simulink model "design"  (Simulink 8.4)
settings: Solver=ode23tb  StartTime=0.0  StopTime=1  MaxStep=0.0001  MinStep=0.00001  RelTol=1e-3
libraries: powerlib x63, simulink x12, powerlib_meascontrol x8, RCTblocks x2
settings Model: Creator=SELVA  LastModifiedBy=SELVA  CovSFcnEnable=on
settings DataIOCC: SignalLoggingSaveFormat=Dataset
settings OptimizationCC: ExpressionDepthLimit=128
settings DebuggingCC: UnderspecifiedInitializationDetection=Simplified  MergeDetectMultiDrivingBlocksExec=error  SolverPrmCheckMsg=none  FcnCallInpInsideContextMsg=EnableAllAsError  FrameProcessingCompatibilityMsg=error  StateNameClashWarn=none
settings GRTTargetCC: CombineOutputUpdateFcns=on  GRTInterface=off

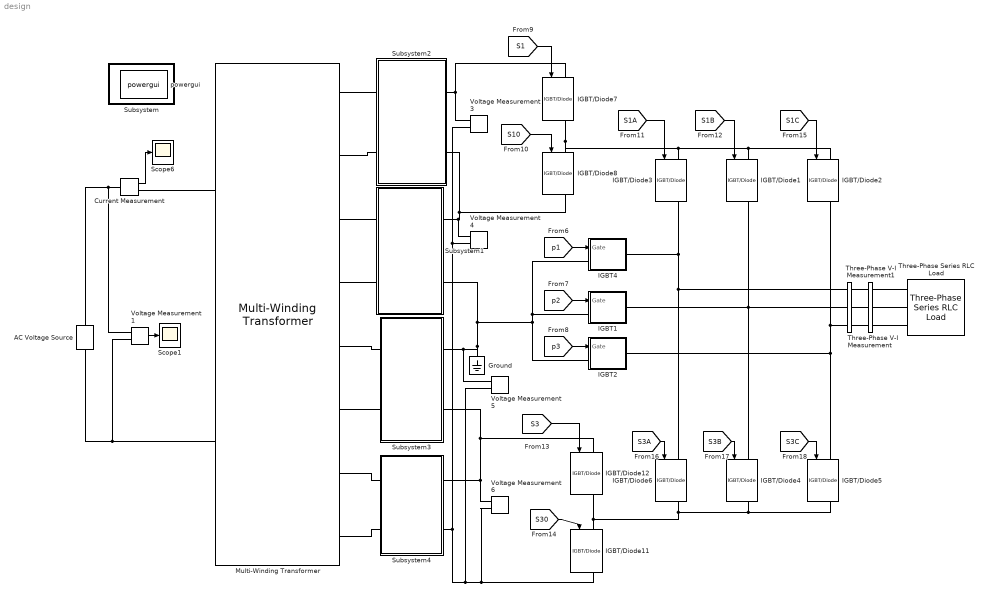
== system design ==
  AC Voltage Source : powerlib/Electrical Sources/AC Voltage Source  Amplitude=325  Phase=0  Frequency=50  SampleTime=0  Measurements=None
  Current Measurement : powerlib/Measurements/Current Measurement  PhasorSimulation=off  OutputType=Complex  PSBequivalent=0
  Ground : powerlib/Elements/Ground  LConnTagsString=a
  IGBT/Diode{1..8,11..12} (10 alike) : powerlib/Power Electronics/IGBT//Diode  Ron=1e-3  Rs=1e5  Cs=inf  Measurements=on
  IGBT1 : Subsystem
  IGBT2 : Subsystem
  IGBT4 : Subsystem
  Multi-Winding Transformer : powerlib/Elements/Multi-Winding Transformer  LeftWindings=1  RightWindings=4  TappedWindings=no taps  NumberOfTaps=2  UNITS=pu  NominalPower=[5000 50]  NominalVoltages="[ 230  115  115 115 115 ]"  WindingResistances="[ 0.005  0.005  0.005  0.005 0.005 ]"  WindingInductances="[ 0.02  0.02  0.02  0.02 0.02 ]"  SetSaturation=on  Rm=50  Lm=50  Saturation=[ 0,0 ; 0.0024,1.2 ; 1.0,1.52 ]  Hysteresis=off  DataFile='hysteresis.mat'  Measurements=Winding currents  MoreParameters=off  BreakLoop=off  DataType=off  InitialFlux=-1.03442051469817  TransfoNumber=1
  Scope1 : Scope
      settings: YMin=3.95  YMax=4.8  SaveName=ScopeData9
  Scope6 : Scope
      settings: YMin=3.95  YMax=4.8  SaveName=ScopeData2
  Subsystem : Subsystem
      mask Display: fprintf('MEASUREMENT \n BLOCK')
  Subsystem1 : Subsystem  mask{r=0, c=1330e-6}
      mask prompts: r "Resistance"; c "Capacitace"
      mask Display: fprintf('Vdc \n RECTIFIER \n WITH \n FILTER')
  Subsystem2 : Subsystem  mask{r=0, c=1330e-6}
      mask prompts: r "Resistance"; c "Capacitace"
      mask Display: fprintf('Vdc \n RECTIFIER \n WITH \n FILTER')
  Subsystem3 : Subsystem  mask{r=0, c=1330e-6}
      mask prompts: r "Resistance"; c "Capacitace"
      mask Display: fprintf('Vdc \n RECTIFIER \n WITH \n FILTER')
  Subsystem4 : Subsystem  mask{r=0, c=1330e-6}
      mask prompts: r "Resistance"; c "Capacitace"
      mask Display: fprintf('Vdc \n RECTIFIER \n WITH \n FILTER')
  Three-Phase Series RLC Load : powerlib/Elements/Three-Phase Series RLC Load  LConnTagsString=A|B|C  Configuration=Y (grounded)  NominalVoltage=400  NominalFrequency=50  ActivePower=500  InductivePower=0  CapacitivePower=0  Measurements=None  LoadType=constant Z
  Three-Phase V-I Measurement : powerlib/Measurements/Three-Phase V-I Measurement  VoltageMeasurement=phase-to-ground  SetLabelV=on  LabelV=Vph  Vpu=off  VpuLL=off  CurrentMeasurement=yes  SetLabelI=on  LabelI=Iab  Ipu=off  Pbase=100e6  Vbase=500e3  OutputType=Complex  PhasorSimulation=off  PSBequivalent=0
  Three-Phase V-I Measurement1 : powerlib/Measurements/Three-Phase V-I Measurement  VoltageMeasurement=phase-to-phase  SetLabelV=on  LabelV=Vl  Vpu=off  VpuLL=off  CurrentMeasurement=yes  SetLabelI=on  LabelI=Iabc  Ipu=off  Pbase=100e6  Vbase=500e3  OutputType=Complex  PhasorSimulation=off  PSBequivalent=0
  Voltage Measurement{1,3..6} (5 alike) : powerlib/Measurements/Voltage Measurement  PhasorSimulation=off  OutputType=Complex  PSBequivalent=0
  powergui : powerlib/powergui  Priority=1  SimulationMode=Discrete  SolverType=Tustin/Backward Euler (TBE)  SampleTime=50e-6  frequency=60  SPID=off  DisableSnubberDevices=off  DisableRonSwitches=off  DisableVfSwitches=off  SwTol=0  DisplayEquations=off  Interpol=off  methode=off  Ts=100  frequencyindice=0  Pbase=100e6  ErrMax=1e-4  Iterations=50  UnitsV=kV  UnitsW=MW  FunctionMessages=off  echomessages=off  HookPort=off  EnableUseOfTLC=off  x0status=blocks  RestoreLinks=warning  ResistiveCurrentMeasurement=off  Frange=[0:2:500]  Ylog=off  Xlog=off  ShowGrid=off  save=off  variable=ZData  structure=ScopeData1  ZoomFFT=off  StartTime=0.5  cycles=1  DisplayStyle=1  fundamental=50  FreqAxis=off  MaxFrequency=1000  frequencyindicesteady=1  RmsSteady=1  display=off
  wires:
  [S3C] -> IGBT/Diode5/1
  [S1A] -> IGBT/Diode3/1
  [S1B] -> IGBT/Diode1/1
  [S1C] -> IGBT/Diode2/1
  [S3A] -> IGBT/Diode6/1
  [S3B] -> IGBT/Diode4/1
  Current Measurement/1 -> Scope6/1
  [S3] -> IGBT/Diode12/1
  [p2] -> IGBT1/1(Gate)
  [p3] -> IGBT2/1(Gate)
  [p1] -> IGBT4/1(Gate)
  [S10] -> IGBT/Diode8/1
  [S1] -> IGBT/Diode7/1
  [S30] -> IGBT/Diode11/1
  Voltage Measurement1/1 -> Scope1/1
  connections:
  Three-Phase V-I Measurement/LConn1 -- IGBT4/RConn1 -- IGBT/Diode3/RConn1 -- IGBT/Diode6/LConn1
  IGBT/Diode3/LConn1 -- IGBT/Diode7/RConn1 -- IGBT/Diode8/LConn1 -- IGBT/Diode2/LConn1 -- IGBT/Diode1/LConn1
  Three-Phase V-I Measurement1/LConn2 -- Three-Phase V-I Measurement/RConn2
  Three-Phase V-I Measurement1/LConn1 -- Three-Phase V-I Measurement/RConn1
  Three-Phase V-I Measurement1/LConn3 -- Three-Phase V-I Measurement/RConn3
  Three-Phase Series RLC Load/LConn2 -- Three-Phase V-I Measurement1/RConn2
  Three-Phase Series RLC Load/LConn1 -- Three-Phase V-I Measurement1/RConn1
  Three-Phase V-I Measurement1/RConn3 -- Three-Phase Series RLC Load/LConn3
  Subsystem2/LConn2 -- Multi-Winding Transformer/RConn2
  Subsystem1/LConn2 -- Multi-Winding Transformer/RConn4
  Subsystem3/LConn1 -- Multi-Winding Transformer/RConn5
  Subsystem1/LConn1 -- Multi-Winding Transformer/RConn3
  Subsystem3/LConn2 -- Multi-Winding Transformer/RConn6
  Subsystem2/LConn1 -- Multi-Winding Transformer/RConn1
  AC Voltage Source/LConn1 -- Voltage Measurement1/LConn2 -- Multi-Winding Transformer/LConn2
  Current Measurement/LConn1 -- Voltage Measurement1/LConn1 -- AC Voltage Source/RConn1
  Current Measurement/RConn1 -- Multi-Winding Transformer/LConn1
  IGBT/Diode4/RConn1 -- IGBT/Diode11/LConn1 -- IGBT/Diode12/RConn1 -- IGBT/Diode6/RConn1 -- IGBT/Diode5/RConn1
  IGBT/Diode12/LConn1 -- Voltage Measurement6/LConn1 -- Subsystem4/RConn1 -- Subsystem3/RConn2
  Subsystem2/RConn2 -- Voltage Measurement4/LConn1 -- Subsystem1/RConn1 -- IGBT/Diode8/RConn1
  IGBT/Diode2/RConn1 -- IGBT/Diode5/LConn1 -- IGBT2/RConn1 -- Three-Phase V-I Measurement/LConn3
  Three-Phase V-I Measurement/LConn2 -- IGBT/Diode4/LConn1 -- IGBT1/RConn1 -- IGBT/Diode1/RConn1
  Subsystem4/RConn2 -- Voltage Measurement4/LConn2 -- Voltage Measurement3/LConn2 -- Voltage Measurement5/LConn2 -- Voltage Measurement6/LConn2 -- IGBT/Diode11/RConn1
  Subsystem2/RConn1 -- Voltage Measurement3/LConn1 -- IGBT/Diode7/LConn1
  Multi-Winding Transformer/RConn8 -- Subsystem4/LConn2
  Multi-Winding Transformer/RConn7 -- Subsystem4/LConn1
  IGBT4/LConn1 -- IGBT1/LConn1 -- IGBT2/LConn1 -- Voltage Measurement5/LConn1 -- Subsystem3/RConn1 -- Ground/LConn1 -- Subsystem1/RConn2

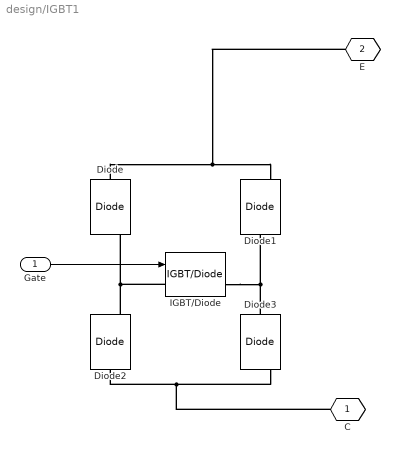
== system design/IGBT1 ==
  Gate : Inport
  Diode{,1..3} (4 alike) : powerlib/Power Electronics/Diode  Ron=0.001  Lon=0  Vf=0.8  IC=0  UseSnubber=off  Rs=500  Cs=250e-9  Measurements=on
  IGBT/Diode : powerlib/Power Electronics/IGBT//Diode  Ron=1e-3  Rs=1e5  Cs=inf  Measurements=on
  C : PMIOPort  Port=1  Side=Left
  E : PMIOPort  Port=2  Side=Right
  wires:
  Gate/1 -> IGBT/Diode/1
  connections:
  E/RConn1 -- Diode/LConn1 -- Diode1/RConn1
  C/RConn1 -- Diode3/RConn1 -- Diode2/LConn1
  IGBT/Diode/RConn1 -- Diode3/LConn1 -- Diode1/LConn1
  IGBT/Diode/LConn1 -- Diode2/RConn1 -- Diode/RConn1

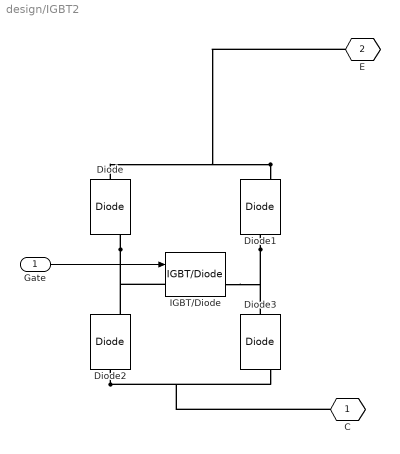
== system design/IGBT2 ==
  Gate : Inport
  Diode{,1..3} (4 alike) : powerlib/Power Electronics/Diode  Ron=0.001  Lon=0  Vf=0.8  IC=0  UseSnubber=off  Rs=500  Cs=250e-9  Measurements=on
  IGBT/Diode : powerlib/Power Electronics/IGBT//Diode  Ron=1e-3  Rs=1e5  Cs=inf  Measurements=on
  C : PMIOPort  Port=1  Side=Left
  E : PMIOPort  Port=2  Side=Right
  wires:
  Gate/1 -> IGBT/Diode/1
  connections:
  Diode/RConn1 -- Diode2/RConn1 -- IGBT/Diode/LConn1
  Diode1/LConn1 -- Diode3/LConn1 -- IGBT/Diode/RConn1
  Diode2/LConn1 -- Diode3/RConn1 -- C/RConn1
  Diode1/RConn1 -- Diode/LConn1 -- E/RConn1

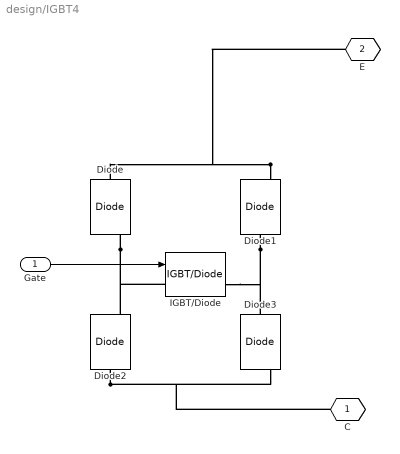
== system design/IGBT4 ==
  Gate : Inport
  Diode{,1..3} (4 alike) : powerlib/Power Electronics/Diode  Ron=0.001  Lon=0  Vf=0.8  IC=0  UseSnubber=off  Rs=500  Cs=250e-9  Measurements=on
  IGBT/Diode : powerlib/Power Electronics/IGBT//Diode  Ron=1e-3  Rs=1e5  Cs=inf  Measurements=on
  C : PMIOPort  Port=1  Side=Left
  E : PMIOPort  Port=2  Side=Right
  wires:
  Gate/1 -> IGBT/Diode/1
  connections:
  Diode/RConn1 -- Diode2/RConn1 -- IGBT/Diode/LConn1
  Diode1/LConn1 -- Diode3/LConn1 -- IGBT/Diode/RConn1
  Diode2/LConn1 -- Diode3/RConn1 -- C/RConn1
  Diode1/RConn1 -- Diode/LConn1 -- E/RConn1

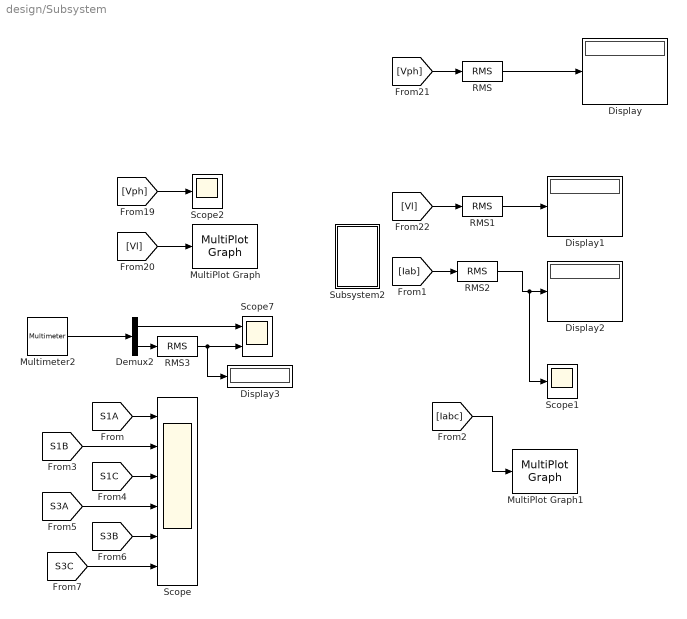
== system design/Subsystem ==
  Demux2 : Demux  Outputs=2
  Display{,1..3} (4 alike) : Display
  MultiPlot Graph : RCTblocks/MultiPlot Graph  Tag=MultiPlot  tmin=0  tmax=20  ymin=-1  ymax=1  Tsamp=-1  vnamesave=multisimout
  MultiPlot Graph1 : RCTblocks/MultiPlot Graph  Tag=MultiPlot  tmin=0  tmax=20  ymin=-1  ymax=1  Tsamp=-1  vnamesave=multisimout1
  Multimeter2 : powerlib/Measurements/Multimeter  PhasorSimulation=off  OutputType=Complex  sel=[11 10]  L=14  Gain=[1 1]  yselected={'I_RightWinding_1: Multi-Winding Transformer','I_LeftWinding_1: Multi-Winding Transformer'};  PSBOutputType=1  PSBequivalent=0  AxesSetting=[0,0.1,-100,100]  Display=0  SavedBlockNames=-11
  RMS{,1..3} (4 alike) : powerlib_meascontrol/Measurements/RMS  TrueRMS=on  Freq=50  RMSInit=0  Ts=0
  Scope : Scope  NumInputPorts=6
      settings: TimeRange=1  YMin=0.7416015625000001~0~0~0~0~0  YMax=0.8755859375~1~1~1~1~1  SaveName=ScopeData7
  Scope1 : Scope
      settings: YMin=0.968  YMax=0.987
  Scope2 : Scope
      settings: YMin=-350  YMax=350
  Scope7 : Scope  NumInputPorts=2
      settings: YMin=-175~-350  YMax=175~350  SaveName=ScopeData6
  Subsystem2 : Subsystem  mask{fc=1000, m=1}
      mask prompts: fc "Switching frequency"; m "modulation index"
  wires:
  [Vph] -> Scope2/1
  [Vl] -> MultiPlot Graph/1
  RMS/1 -> Display/1
  [Vph] -> RMS/1
  RMS1/1 -> Display1/1
  [Vl] -> RMS1/1
  [Iab] -> RMS2/1
  RMS2/1 -> Scope1/1, Display2/1
  [Iabc] -> MultiPlot Graph1/1
  Multimeter2/1 -> Demux2/1
  Demux2/1 -> Scope7/1
  [S1A] -> Scope/1
  [S1B] -> Scope/2
  [S1C] -> Scope/3
  [S3A] -> Scope/4
  [S3B] -> Scope/5
  [S3C] -> Scope/6
  Demux2/2 -> RMS3/1
  RMS3/1 -> Display3/1, Scope7/2

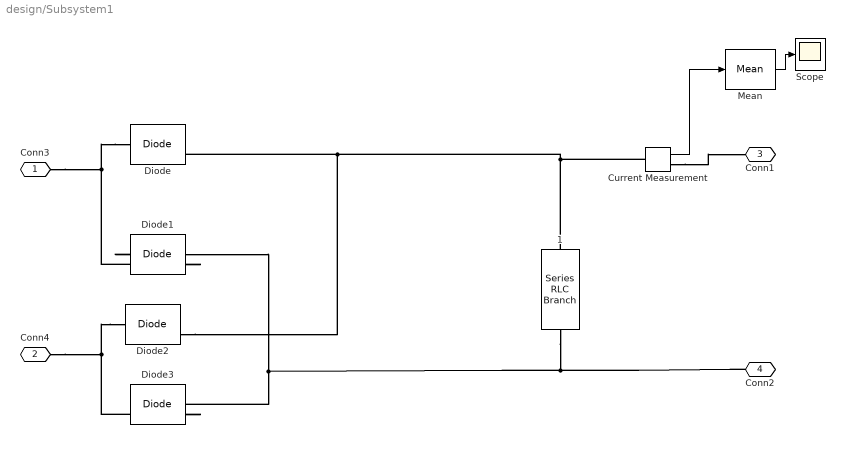
== system design/Subsystem1 ==
  1 : powerlib/Elements/Series RLC Branch  LConnTagsString=__new0  RConnTagsString=__new0  BranchType=C  Resistance=r  Inductance=1e-3  SetiL0=off  InitialCurrent=0  Capacitance=c  Setx0=off  InitialVoltage=0  Measurements=Branch voltage and current
  Current Measurement : powerlib/Measurements/Current Measurement  PhasorSimulation=off  OutputType=Complex  PSBequivalent=0
  Diode{,1..3} (4 alike) : powerlib/Power Electronics/Diode  Ron=0.001  Lon=0  Vf=0.8  IC=0  UseSnubber=off  Rs=500  Cs=250e-9  Measurements=on
  Mean : powerlib_meascontrol/Measurements/Mean  Freq=50  Vinit=0  Ts=0
  Scope : Scope
      settings: YMin=0.6175  YMax=0.67  SaveName=ScopeData8
  Conn3 : PMIOPort  Port=1  Side=Left
  Conn4 : PMIOPort  Port=2  Side=Left
  Conn1 : PMIOPort  Port=3  Side=Right
  Conn2 : PMIOPort  Port=4  Side=Right
  wires:
  Mean/1 -> Scope/1
  Current Measurement/1 -> Mean/1
  connections:
  Current Measurement/RConn1 -- Conn1/RConn1
  Diode/RConn1 -- 1/LConn1 -- Current Measurement/LConn1 -- Diode2/RConn1
  Diode2/LConn1 -- Conn4/RConn1 -- Diode3/RConn1
  Diode/LConn1 -- Conn3/RConn1 -- Diode1/RConn1
  Diode1/LConn1 -- 1/RConn1 -- Conn2/RConn1 -- Diode3/LConn1

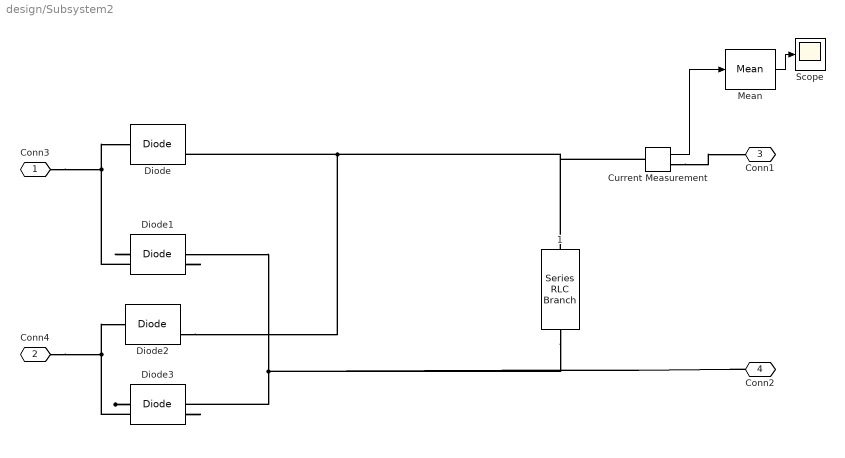
== system design/Subsystem2 ==
  1 : powerlib/Elements/Series RLC Branch  LConnTagsString=__new0  RConnTagsString=__new0  BranchType=C  Resistance=r  Inductance=1e-3  SetiL0=off  InitialCurrent=0  Capacitance=c  Setx0=off  InitialVoltage=0  Measurements=Branch voltage and current
  Current Measurement : powerlib/Measurements/Current Measurement  PhasorSimulation=off  OutputType=Complex  PSBequivalent=0
  Diode{,1..3} (4 alike) : powerlib/Power Electronics/Diode  Ron=0.001  Lon=0  Vf=0.8  IC=0  UseSnubber=off  Rs=500  Cs=250e-9  Measurements=on
  Mean : powerlib_meascontrol/Measurements/Mean  Freq=50  Vinit=0  Ts=0
  Scope : Scope
      settings: YMin=0.6175  YMax=0.67  SaveName=ScopeData8
  Conn3 : PMIOPort  Port=1  Side=Left
  Conn4 : PMIOPort  Port=2  Side=Left
  Conn1 : PMIOPort  Port=3  Side=Right
  Conn2 : PMIOPort  Port=4  Side=Right
  wires:
  Current Measurement/1 -> Mean/1
  Mean/1 -> Scope/1
  connections:
  Diode3/LConn1 -- Conn2/RConn1 -- 1/RConn1 -- Diode1/LConn1
  Diode1/RConn1 -- Conn3/RConn1 -- Diode/LConn1
  Diode3/RConn1 -- Conn4/RConn1 -- Diode2/LConn1
  Diode2/RConn1 -- Current Measurement/LConn1 -- 1/LConn1 -- Diode/RConn1
  Current Measurement/RConn1 -- Conn1/RConn1

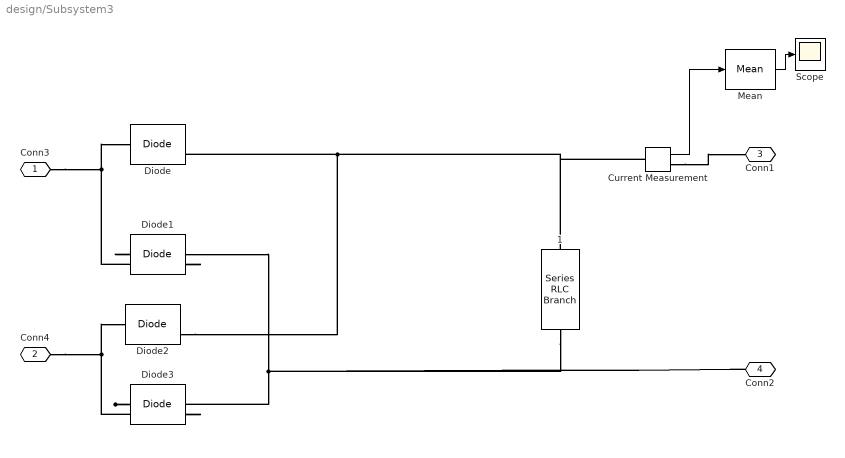
== system design/Subsystem3 ==
  1 : powerlib/Elements/Series RLC Branch  LConnTagsString=__new0  RConnTagsString=__new0  BranchType=C  Resistance=r  Inductance=1e-3  SetiL0=off  InitialCurrent=0  Capacitance=c  Setx0=off  InitialVoltage=0  Measurements=Branch voltage and current
  Current Measurement : powerlib/Measurements/Current Measurement  PhasorSimulation=off  OutputType=Complex  PSBequivalent=0
  Diode{,1..3} (4 alike) : powerlib/Power Electronics/Diode  Ron=0.001  Lon=0  Vf=0.8  IC=0  UseSnubber=off  Rs=500  Cs=250e-9  Measurements=on
  Mean : powerlib_meascontrol/Measurements/Mean  Freq=50  Vinit=0  Ts=0
  Scope : Scope
      settings: YMin=0.6175  YMax=0.67  SaveName=ScopeData8
  Conn3 : PMIOPort  Port=1  Side=Left
  Conn4 : PMIOPort  Port=2  Side=Left
  Conn1 : PMIOPort  Port=3  Side=Right
  Conn2 : PMIOPort  Port=4  Side=Right
  wires:
  Current Measurement/1 -> Mean/1
  Mean/1 -> Scope/1
  connections:
  Diode3/LConn1 -- Conn2/RConn1 -- 1/RConn1 -- Diode1/LConn1
  Diode1/RConn1 -- Conn3/RConn1 -- Diode/LConn1
  Diode3/RConn1 -- Conn4/RConn1 -- Diode2/LConn1
  Diode2/RConn1 -- Current Measurement/LConn1 -- 1/LConn1 -- Diode/RConn1
  Current Measurement/RConn1 -- Conn1/RConn1

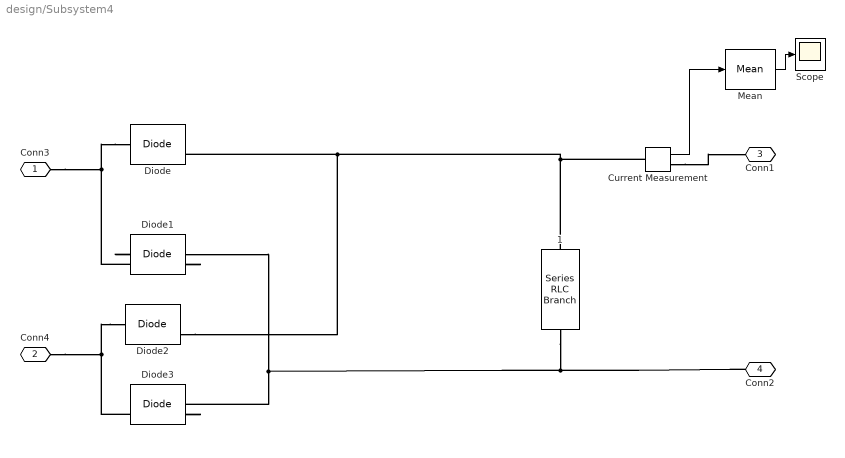
== system design/Subsystem4 ==
  1 : powerlib/Elements/Series RLC Branch  LConnTagsString=__new0  RConnTagsString=__new0  BranchType=C  Resistance=r  Inductance=1e-3  SetiL0=off  InitialCurrent=0  Capacitance=c  Setx0=off  InitialVoltage=0  Measurements=Branch voltage and current
  Current Measurement : powerlib/Measurements/Current Measurement  PhasorSimulation=off  OutputType=Complex  PSBequivalent=0
  Diode{,1..3} (4 alike) : powerlib/Power Electronics/Diode  Ron=0.001  Lon=0  Vf=0.8  IC=0  UseSnubber=off  Rs=500  Cs=250e-9  Measurements=on
  Mean : powerlib_meascontrol/Measurements/Mean  Freq=50  Vinit=0  Ts=0
  Scope : Scope
      settings: YMin=0.6175  YMax=0.67  SaveName=ScopeData8
  Conn3 : PMIOPort  Port=1  Side=Left
  Conn4 : PMIOPort  Port=2  Side=Left
  Conn1 : PMIOPort  Port=3  Side=Right
  Conn2 : PMIOPort  Port=4  Side=Right
  wires:
  Mean/1 -> Scope/1
  Current Measurement/1 -> Mean/1
  connections:
  Current Measurement/RConn1 -- Conn1/RConn1
  Diode/RConn1 -- 1/LConn1 -- Current Measurement/LConn1 -- Diode2/RConn1
  Diode2/LConn1 -- Conn4/RConn1 -- Diode3/RConn1
  Diode/LConn1 -- Conn3/RConn1 -- Diode1/RConn1
  Diode1/LConn1 -- 1/RConn1 -- Conn2/RConn1 -- Diode3/LConn1

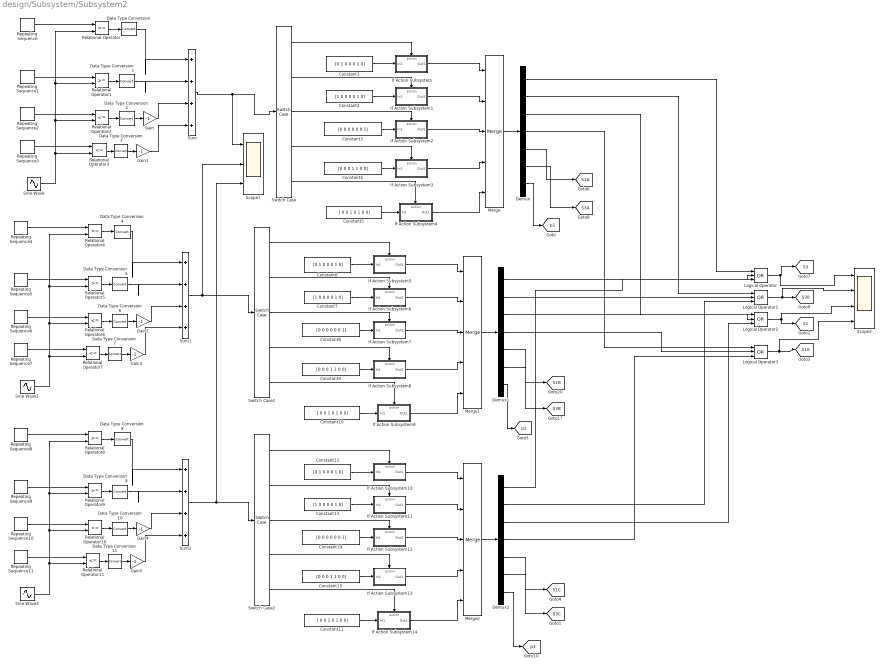
== system design/Subsystem/Subsystem2 ==
  Constant1 : Constant  Value=[0 1 0 0 0 1 0]
  Constant10 : Constant  Value=[ 0 0 1 0 1 0 0]
  Constant11 : Constant  Value=[ 0 0 1 0 1 0 0]
  Constant12 : Constant  Value=[0 1 0 0 0 1 0]
  Constant13 : Constant  Value=[1 0 0 0 0 1 0]
  Constant14 : Constant  Value=[0 0 0 0 0 0 1]
  Constant15 : Constant  Value=[0 0 0 1 1 0 0]
  Constant2 : Constant  Value=[1 0 0 0 0 1 0]
  Constant3 : Constant  Value=[0 0 0 0 0 0 1]
  Constant4 : Constant  Value=[0 0 0 1 1 0 0]
  Constant5 : Constant  Value=[ 0 0 1 0 1 0 0]
  Constant6 : Constant  Value=[0 1 0 0 0 1 0]
  Constant7 : Constant  Value=[1 0 0 0 0 1 0]
  Constant8 : Constant  Value=[0 0 0 0 0 0 1]
  Constant9 : Constant  Value=[0 0 0 1 1 0 0]
  Data Type Conversion{,1..11} (12 alike) : DataTypeConversion
  Demux : Demux  Outputs=7
  Demux1 : Demux  Outputs=7
  Demux2 : Demux  Outputs=7
  Gain{,1..5} (6 alike) : Gain  Gain=-1
  If Action Subsystem : Subsystem  TreatAsAtomicUnit=on
  If Action Subsystem1 : Subsystem  TreatAsAtomicUnit=on
  If Action Subsystem10 : Subsystem  TreatAsAtomicUnit=on
  If Action Subsystem11 : Subsystem  TreatAsAtomicUnit=on
  If Action Subsystem12 : Subsystem  TreatAsAtomicUnit=on
  If Action Subsystem13 : Subsystem  TreatAsAtomicUnit=on
  If Action Subsystem14 : Subsystem  TreatAsAtomicUnit=on
  If Action Subsystem2 : Subsystem  TreatAsAtomicUnit=on
  If Action Subsystem3 : Subsystem  TreatAsAtomicUnit=on
  If Action Subsystem4 : Subsystem  TreatAsAtomicUnit=on
  If Action Subsystem5 : Subsystem  TreatAsAtomicUnit=on
  If Action Subsystem6 : Subsystem  TreatAsAtomicUnit=on
  If Action Subsystem7 : Subsystem  TreatAsAtomicUnit=on
  If Action Subsystem8 : Subsystem  TreatAsAtomicUnit=on
  If Action Subsystem9 : Subsystem  TreatAsAtomicUnit=on
  Logical Operator{,1..3} (4 alike) : Logic  Operator=OR  Inputs=3  AllPortsSameDT=off  OutDataTypeStr=boolean
  Merge : Merge  Inputs=5
  Merge1 : Merge  Inputs=5
  Merge2 : Merge  Inputs=5
  Relational Operator{,1,4..5,8..9} (6 alike) : RelationalOperator  OutDataTypeStr=boolean
  Relational Operator{2..3,6..7,10..11} (6 alike) : RelationalOperator  Operator=<=  OutDataTypeStr=boolean
  Repeating Sequence : simulink/Sources/Repeating Sequence  rep_seq_t="[0 (1/fc)/2  (1/fc)]"  rep_seq_y=[1 2 1]
  Repeating Sequence1 : simulink/Sources/Repeating Sequence  rep_seq_t="[0 (1/fc)/2  (1/fc)]"  rep_seq_y=[1 0 1]
  Repeating Sequence10 : simulink/Sources/Repeating Sequence  rep_seq_t="[0 (1/fc)/2  (1/fc)]"  rep_seq_y=[-1 0 -1]
  Repeating Sequence11 : simulink/Sources/Repeating Sequence  rep_seq_t="[0 (1/fc)/2  (1/fc)]"  rep_seq_y=[-1 -2 -1]
  Repeating Sequence2 : simulink/Sources/Repeating Sequence  rep_seq_t="[0 (1/fc)/2  (1/fc)]"  rep_seq_y=[-1 0 -1]
  Repeating Sequence3 : simulink/Sources/Repeating Sequence  rep_seq_t="[0 (1/fc)/2  (1/fc)]"  rep_seq_y=[-1 -2 -1]
  Repeating Sequence4 : simulink/Sources/Repeating Sequence  rep_seq_t="[0 (1/fc)/2  (1/fc)]"  rep_seq_y=[1 2 1]
  Repeating Sequence5 : simulink/Sources/Repeating Sequence  rep_seq_t="[0 (1/fc)/2  (1/fc)]"  rep_seq_y=[1 0 1]
  Repeating Sequence6 : simulink/Sources/Repeating Sequence  rep_seq_t="[0 (1/fc)/2  (1/fc)]"  rep_seq_y=[-1 0 -1]
  Repeating Sequence7 : simulink/Sources/Repeating Sequence  rep_seq_t="[0 (1/fc)/2  (1/fc)]"  rep_seq_y=[-1 -2 -1]
  Repeating Sequence8 : simulink/Sources/Repeating Sequence  rep_seq_t="[0 (1/fc)/2  (1/fc)]"  rep_seq_y=[1 2 1]
  Repeating Sequence9 : simulink/Sources/Repeating Sequence  rep_seq_t="[0 (1/fc)/2  (1/fc)]"  rep_seq_y=[1 0 1]
  Scope1 : Scope  NumInputPorts=3
      settings: YMin=-250~-5~-5  YMax=250~5~5  SaveName=ScopeData4
  Scope2 : Scope  NumInputPorts=4
      settings: YMin=-250~-5~-5~-5  YMax=250~5~5~5
  Sine Wave : Sin  Amplitude=2*m  Frequency=2*pi*50  SampleTime=0
  Sine Wave1 : Sin  Amplitude=2*m  Frequency=2*pi*50  Phase=120*pi/180  SampleTime=0
  Sine Wave2 : Sin  Amplitude=2*m  Frequency=2*pi*50  Phase=240*pi/180  SampleTime=0
  Sum : Sum  Inputs=|++++
  Sum1 : Sum  Inputs=|++++
  Sum2 : Sum  Inputs=|++++
  Switch Case : SwitchCase  CaseConditions={-2 -1 0 1 2}  ShowDefaultCase=off
  Switch Case1 : SwitchCase  CaseConditions={-2 -1 0 1 2}  ShowDefaultCase=off
  Switch Case2 : SwitchCase  CaseConditions={-2 -1 0 1 2}  ShowDefaultCase=off
  tag scope: S10=global, S1=global, S1A=global, S1B=global, S1C=global, S30=global, S3=global, S3A=global, S3B=global, S3C=global, p1=global, p2=global, p3=global
  wires:
  Logical Operator2/1 -> Scope2/3, [S1]
  Demux2/4 -> Logical Operator3/3
  Demux2/3 -> Logical Operator2/3
  Demux2/2 -> Logical Operator1/3
  Demux2/1 -> Logical Operator/3
  Demux2/6 -> [S3C]
  Demux2/5 -> [S1C]
  Sum2/1 -> Switch Case2/1, Scope1/3
  Merge2/1 -> Demux2/1
  If Action Subsystem14/1(Out1) -> Merge2/5
  If Action Subsystem13/1(Out1) -> Merge2/4
  If Action Subsystem12/1(Out1) -> Merge2/3
  If Action Subsystem11/1(Out1) -> Merge2/2
  If Action Subsystem10/1(Out1) -> Merge2/1
  Constant11/1 -> If Action Subsystem14/1(In1)
  Constant15/1 -> If Action Subsystem13/1(In1)
  Constant14/1 -> If Action Subsystem12/1(In1)
  Constant13/1 -> If Action Subsystem11/1(In1)
  Constant12/1 -> If Action Subsystem10/1(In1)
  Switch Case2/1 -> If Action Subsystem10/Action
  Switch Case2/2 -> If Action Subsystem11/Action
  Switch Case2/3 -> If Action Subsystem12/Action
  Switch Case2/4 -> If Action Subsystem13/Action
  Switch Case2/5 -> If Action Subsystem14/Action
  Logical Operator3/1 -> [S10], Scope2/4
  Logical Operator1/1 -> [S30], Scope2/2
  Logical Operator/1 -> [S3], Scope2/1
  Demux1/4 -> Logical Operator3/2
  Demux1/3 -> Logical Operator2/2
  Demux/4 -> Logical Operator3/1
  Demux/3 -> Logical Operator2/1
  Demux1/2 -> Logical Operator1/2
  Demux/2 -> Logical Operator1/1
  Demux1/1 -> Logical Operator/2
  Demux/1 -> Logical Operator/1
  Demux1/6 -> [S3B]
  Demux1/5 -> [S1B]
  Sum1/1 -> Switch Case1/1, Scope1/2
  Merge1/1 -> Demux1/1
  If Action Subsystem9/1(Out1) -> Merge1/5
  If Action Subsystem8/1(Out1) -> Merge1/4
  If Action Subsystem7/1(Out1) -> Merge1/3
  If Action Subsystem6/1(Out1) -> Merge1/2
  If Action Subsystem5/1(Out1) -> Merge1/1
  Constant10/1 -> If Action Subsystem9/1(In1)
  Constant9/1 -> If Action Subsystem8/1(In1)
  Constant8/1 -> If Action Subsystem7/1(In1)
  Constant7/1 -> If Action Subsystem6/1(In1)
  Constant6/1 -> If Action Subsystem5/1(In1)
  Switch Case1/1 -> If Action Subsystem5/Action
  Switch Case1/2 -> If Action Subsystem6/Action
  Switch Case1/3 -> If Action Subsystem7/Action
  Switch Case1/4 -> If Action Subsystem8/Action
  Switch Case1/5 -> If Action Subsystem9/Action
  Demux/5 -> [S1A]
  Demux/6 -> [S3A]
  Data Type Conversion11/1 -> Gain5/1
  Data Type Conversion10/1 -> Gain4/1
  Data Type Conversion9/1 -> Sum2/2
  Data Type Conversion8/1 -> Sum2/1
  Relational Operator11/1 -> Data Type Conversion11/1
  Relational Operator10/1 -> Data Type Conversion10/1
  Sine Wave2/1 -> Relational Operator11/2, Relational Operator10/2, Relational Operator8/2, Relational Operator9/2
  Repeating Sequence11/1 -> Relational Operator11/1
  Repeating Sequence10/1 -> Relational Operator10/1
  Repeating Sequence9/1 -> Relational Operator9/1
  Repeating Sequence8/1 -> Relational Operator8/1
  Gain5/1 -> Sum2/4
  Gain4/1 -> Sum2/3
  Relational Operator9/1 -> Data Type Conversion9/1
  Relational Operator8/1 -> Data Type Conversion8/1
  Data Type Conversion7/1 -> Gain3/1
  Data Type Conversion6/1 -> Gain2/1
  Data Type Conversion5/1 -> Sum1/2
  Data Type Conversion4/1 -> Sum1/1
  Relational Operator7/1 -> Data Type Conversion7/1
  Relational Operator6/1 -> Data Type Conversion6/1
  Sine Wave1/1 -> Relational Operator5/2, Relational Operator4/2, Relational Operator6/2, Relational Operator7/2
  Repeating Sequence7/1 -> Relational Operator7/1
  Repeating Sequence6/1 -> Relational Operator6/1
  Repeating Sequence5/1 -> Relational Operator5/1
  Repeating Sequence4/1 -> Relational Operator4/1
  Gain3/1 -> Sum1/4
  Gain2/1 -> Sum1/3
  Relational Operator5/1 -> Data Type Conversion5/1
  Relational Operator4/1 -> Data Type Conversion4/1
  Data Type Conversion3/1 -> Gain1/1
  Data Type Conversion2/1 -> Gain/1
  Data Type Conversion1/1 -> Sum/2
  Data Type Conversion/1 -> Sum/1
  Relational Operator3/1 -> Data Type Conversion3/1
  Relational Operator2/1 -> Data Type Conversion2/1
  Sine Wave/1 -> Relational Operator3/2, Relational Operator2/2, Relational Operator/2, Relational Operator1/2
  Repeating Sequence3/1 -> Relational Operator3/1
  Repeating Sequence2/1 -> Relational Operator2/1
  Repeating Sequence1/1 -> Relational Operator1/1
  Repeating Sequence/1 -> Relational Operator/1
  Sum/1 -> Switch Case/1, Scope1/1
  Gain1/1 -> Sum/4
  Gain/1 -> Sum/3
  Relational Operator1/1 -> Data Type Conversion1/1
  Relational Operator/1 -> Data Type Conversion/1
  Merge/1 -> Demux/1
  If Action Subsystem4/1(Out1) -> Merge/5
  If Action Subsystem3/1(Out1) -> Merge/4
  If Action Subsystem2/1(Out1) -> Merge/3
  If Action Subsystem1/1(Out1) -> Merge/2
  If Action Subsystem/1(Out1) -> Merge/1
  Constant5/1 -> If Action Subsystem4/1(In1)
  Constant4/1 -> If Action Subsystem3/1(In1)
  Constant3/1 -> If Action Subsystem2/1(In1)
  Constant2/1 -> If Action Subsystem1/1(In1)
  Constant1/1 -> If Action Subsystem/1(In1)
  Switch Case/1 -> If Action Subsystem/Action
  Switch Case/2 -> If Action Subsystem1/Action
  Switch Case/3 -> If Action Subsystem2/Action
  Switch Case/4 -> If Action Subsystem3/Action
  Switch Case/5 -> If Action Subsystem4/Action
  Demux/7 -> [p1]
  Demux1/7 -> [p2]
  Demux2/7 -> [p3]

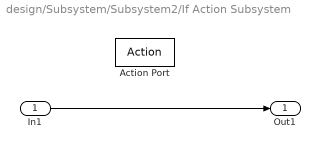
== system design/Subsystem/Subsystem2/If Action Subsystem ==
  In1 : Inport
  Action Port : ActionPort  ActionType=case
  Out1 : Outport
  wires:
  In1/1 -> Out1/1

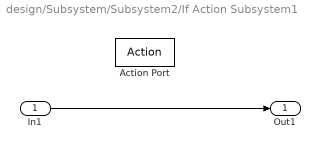
== system design/Subsystem/Subsystem2/If Action Subsystem1 ==
  In1 : Inport
  Action Port : ActionPort  ActionType=case
  Out1 : Outport
  wires:
  In1/1 -> Out1/1

== system design/Subsystem/Subsystem2/If Action Subsystem10 ==
  In1 : Inport
  Action Port : ActionPort  ActionType=case
  Out1 : Outport
  wires:
  In1/1 -> Out1/1

== system design/Subsystem/Subsystem2/If Action Subsystem11 ==
  In1 : Inport
  Action Port : ActionPort  ActionType=case
  Out1 : Outport
  wires:
  In1/1 -> Out1/1

== system design/Subsystem/Subsystem2/If Action Subsystem12 ==
  In1 : Inport
  Action Port : ActionPort  ActionType=case
  Out1 : Outport
  wires:
  In1/1 -> Out1/1

== system design/Subsystem/Subsystem2/If Action Subsystem13 ==
  In1 : Inport
  Action Port : ActionPort  ActionType=case
  Out1 : Outport
  wires:
  In1/1 -> Out1/1

== system design/Subsystem/Subsystem2/If Action Subsystem14 ==
  In1 : Inport
  Action Port : ActionPort  ActionType=case
  Out1 : Outport
  wires:
  In1/1 -> Out1/1

== system design/Subsystem/Subsystem2/If Action Subsystem2 ==
  In1 : Inport
  Action Port : ActionPort  ActionType=case
  Out1 : Outport
  wires:
  In1/1 -> Out1/1

== system design/Subsystem/Subsystem2/If Action Subsystem3 ==
  In1 : Inport
  Action Port : ActionPort  ActionType=case
  Out1 : Outport
  wires:
  In1/1 -> Out1/1

== system design/Subsystem/Subsystem2/If Action Subsystem4 ==
  In1 : Inport
  Action Port : ActionPort  ActionType=case
  Out1 : Outport
  wires:
  In1/1 -> Out1/1

== system design/Subsystem/Subsystem2/If Action Subsystem5 ==
  In1 : Inport
  Action Port : ActionPort  ActionType=case
  Out1 : Outport
  wires:
  In1/1 -> Out1/1

== system design/Subsystem/Subsystem2/If Action Subsystem6 ==
  In1 : Inport
  Action Port : ActionPort  ActionType=case
  Out1 : Outport
  wires:
  In1/1 -> Out1/1

== system design/Subsystem/Subsystem2/If Action Subsystem7 ==
  In1 : Inport
  Action Port : ActionPort  ActionType=case
  Out1 : Outport
  wires:
  In1/1 -> Out1/1

== system design/Subsystem/Subsystem2/If Action Subsystem8 ==
  In1 : Inport
  Action Port : ActionPort  ActionType=case
  Out1 : Outport
  wires:
  In1/1 -> Out1/1

== system design/Subsystem/Subsystem2/If Action Subsystem9 ==
  In1 : Inport
  Action Port : ActionPort  ActionType=case
  Out1 : Outport
  wires:
  In1/1 -> Out1/1
